simulink model "3P Line"  (R2020a)
settings: Solver=VariableStepAuto  StartTime=0.0  StopTime=1.0  RelTol=1e-3
libraries: powerlib x6, powerlib_meascontrol x6
settings Model: Creator=Alisamar  LastModifiedBy=Alisamar

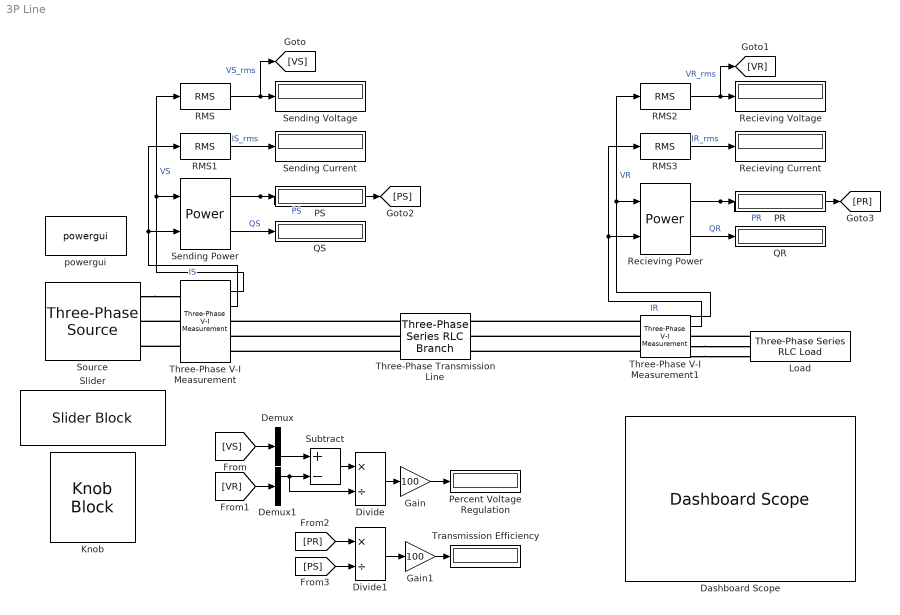
== system 3P Line ==
  Dashboard Scope : DashboardScope
  Demux : Demux  Outputs=3
  Demux1 : Demux  Outputs=3
  Divide : Product  Inputs=*/
  Divide1 : Product  Inputs=*/
  Gain : Gain  Gain=100
  Gain1 : Gain  Gain=100
  Knob : KnobBlock  LabelPosition=Bottom
  Load : powerlib/Elements/Three-Phase Series RLC Load  LConnTagsString=A|B|C  Configuration=Y (grounded)  NominalVoltage=220e3  Vabc=[1e3 1e3 1e3]  Vabcp=[1e3 1e3 1e3]  NominalFrequency=60  UnbalancedPower=off  ActivePower=304.8e6  InductivePower=228.6e6  CapacitivePower=0  Pabc=[10e3 9e3 11e3]  QLabc=[100 90 110]  QCabc=[100 90 110]  Pabcp=[10e3 9e3 11e3]  QLabcp=[100 90 110]  QCabcp=[100 90 110]  Measurements=None  LoadType=constant Z
  PR : Display
      settings: Format=bank
  PS : Display
      settings: Format=bank
  Percent Voltage Regulation : Display
      settings: Format=bank  Decimation=3
  QR : Display
      settings: Format=bank
  QS : Display
      settings: Format=bank
  RMS{,1..3} (4 alike) : powerlib_meascontrol/Measurements/RMS  TrueRMS=on  Freq=60  RMSInit=120  Ts=0
  Recieving Current : Display
      settings: Format=bank  Decimation=3
  Recieving Power : powerlib_meascontrol/Measurements/Power  Freq=60  Vinit=[1, 0]  Iinit=[1, 0]  Ts=0
  Recieving Voltage : Display
      settings: Format=bank  Decimation=3
  Sending Current : Display
      settings: Format=bank  Decimation=3
  Sending Power : powerlib_meascontrol/Measurements/Power  Freq=60  Vinit=[1, 0]  Iinit=[1, 0]  Ts=0
  Sending Voltage : Display
      settings: Format=bank  Decimation=3
  Slider : SliderBlock  LabelPosition=Bottom  ScaleMin=100e3  ScaleMax=750e3
  Source : powerlib/Electrical Sources/Three-Phase Source  InternalConnection=Yg  VoltagePhases=off  Voltage=715899.213576159  PhaseAngle=0  Voltage_phases=[25e3 25e3 25e3]/sqrt(3)  PhaseAngles_phases=[0 -120 +120]  Frequency=80.0908174013686  NonIdealSource=off  SpecifyImpedance=off  Resistance=0.8929  Inductance=16.58e-3  ShortCircuitLevel=100e6  BaseVoltage=25e3  XRratio=7  BusType=swing  Pref=10e3  Qref=0  Prefabc=[10e3, 10e3, 10e3]  Qrefabc=[0, 0, 0]  Qmin=-inf  Qmax=inf
  Subtract : Sum  Inputs=+-
  Three-Phase Transmission Line : powerlib/Elements/Three-Phase Series RLC Branch  LConnTagsString=A|B|C  RConnTagsString=A|B|C  BranchType=RL  Resistance=6  Inductance=0.053052  Capacitance=1e-6  Measurements=None
  Three-Phase V-I Measurement : powerlib/Measurements/Three-Phase V-I Measurement  VoltageMeasurement=phase-to-ground  SetLabelV=off  LabelV=Vabc  Vpu=off  VpuLL=off  CurrentMeasurement=yes  SetLabelI=off  LabelI=Iabc  Ipu=off  Pbase=100e6  Vbase=500e3  OutputType=Complex  PhasorSimulation=off  PSBequivalent=0
  Three-Phase V-I Measurement1 : powerlib/Measurements/Three-Phase V-I Measurement  VoltageMeasurement=phase-to-ground  SetLabelV=off  LabelV=Vabc  Vpu=off  VpuLL=off  CurrentMeasurement=yes  SetLabelI=off  LabelI=Iabc  Ipu=off  Pbase=100e6  Vbase=500e3  OutputType=Complex  PhasorSimulation=off  PSBequivalent=0
  Transmission Efficiency : Display
      settings: Format=bank  Decimation=3
  powergui : powerlib/powergui  Priority=1  SimulationMode=Continuous  SampleTime=50e-6  frequency=60  Iterations=50  frequencyindice=80.0908174013686  Pbase=100e6  ErrMax=1e-4  UnitsV=kV  UnitsW=MW  buscounter=0  FunctionMessages=off  echomessages=off  EnableUseOfTLC=off  CurrentSourceSwitches=off  DisableSnubberDevices=off  DisableRonSwitches=off  DisableVfSwitches=off  DisplayEquations=off  AutomaticDiscreteSolvers=off  SolverType=Tustin/Backward Euler (TBE)  Interpol=off  ExternalGateDelay=off  methode=off  Ts=100  x0status=blocks  SPID=on  SwTol=0  HookPort=off  NonlinearTolerance=1e-4  nMaxIteration=100  ContinueOnMaxIteration=off  RestoreLinks=warning  ResistiveCurrentMeasurement=off  Frange=[0:2:500]  Ylog=off  Xlog=on  ShowGrid=off  save=off  variable=ZData  structure=0  ZoomFFT=off  StartTime=0.0  cycles=1  DisplayStyle=1  fundamental=60  FreqAxis=off  MaxFrequency=1000  frequencyindicesteady=1  RmsSteady=1  display=off
  wires:
  RMS/1 -> [VS], Sending Voltage/1  "VS_rms"
  RMS1/1 -> Sending Current/1  "IS_rms"
  Sending Power/2 -> QS/1  "QS"
  Sending Power/1 -> [PS], PS/1  "PS"
  Three-Phase V-I Measurement/1 -> Sending Power/1, RMS/1  "VS"
  Three-Phase V-I Measurement/2 -> RMS1/1, Sending Power/2  "IS"
  RMS3/1 -> Recieving Current/1  "IR_rms"
  Three-Phase V-I Measurement1/1 -> RMS2/1, Recieving Power/1  "VR"
  Three-Phase V-I Measurement1/2 -> RMS3/1, Recieving Power/2  "IR"
  RMS2/1 -> [VR], Recieving Voltage/1  "VR_rms"
  Recieving Power/1 -> [PR], PR/1  "PR"
  Recieving Power/2 -> QR/1  "QR"
  Demux/3 -> Subtract/1
  Demux1/1 -> Divide/2, Subtract/2
  Subtract/1 -> Divide/1
  Divide/1 -> Gain/1
  [VS] -> Demux/1
  [VR] -> Demux1/1
  Gain/1 -> Percent Voltage Regulation/1
  Gain1/1 -> Transmission Efficiency/1
  Divide1/1 -> Gain1/1
  [PR] -> Divide1/1
  [PS] -> Divide1/2
  connections:
  Source/RConn1 -- Three-Phase V-I Measurement/LConn1
  Three-Phase V-I Measurement/LConn2 -- Source/RConn2
  Three-Phase V-I Measurement/LConn3 -- Source/RConn3
  Three-Phase Transmission Line/LConn1 -- Three-Phase V-I Measurement/RConn1
  Three-Phase Transmission Line/LConn2 -- Three-Phase V-I Measurement/RConn2
  Three-Phase Transmission Line/LConn3 -- Three-Phase V-I Measurement/RConn3
  Three-Phase V-I Measurement1/LConn1 -- Three-Phase Transmission Line/RConn1
  Three-Phase V-I Measurement1/LConn2 -- Three-Phase Transmission Line/RConn2
  Three-Phase V-I Measurement1/LConn3 -- Three-Phase Transmission Line/RConn3
  Three-Phase V-I Measurement1/RConn2 -- Load/LConn2
  Load/LConn1 -- Three-Phase V-I Measurement1/RConn1
  Three-Phase V-I Measurement1/RConn3 -- Load/LConn3
